simulink model "pathFollowingWithObstacleAvoidanceExample"  (R2018a)
settings: Solver=VariableStepAuto  StartTime=0.0  StopTime=inf  FixedStep=0.01  RelTol=1e-3  EnableMultiTasking=on
model workspace (MAT data in the model file):
  SL_ROS_VariableLengthArrays_MaxSizes.CommonInfo.ArrayTruncateAction = 'EmitWarning'
  SL_ROS_VariableLengthArrays_MaxSizes.MsgTypeMap = containers.Map
  SL_ROS_VariableLengthArrays_MaxSizes.MsgTypeMap.serialization.keys = {'sensor_msgs/CompressedImage', 'sensor_msgs/LaserScan'}
  SL_ROS_VariableLengthArrays_MaxSizes.MsgTypeMap.serialization.values{1}(1).PropertyName = 'Data'
  SL_ROS_VariableLengthArrays_MaxSizes.MsgTypeMap.serialization.values{1}(1).DataType = 'uint8'
  SL_ROS_VariableLengthArrays_MaxSizes.MsgTypeMap.serialization.values{1}(1).MaxLength = 10000000
  SL_ROS_VariableLengthArrays_MaxSizes.MsgTypeMap.serialization.values{1}(2).PropertyName = 'Format'
  SL_ROS_VariableLengthArrays_MaxSizes.MsgTypeMap.serialization.values{1}(2).DataType = 'uint8'
  SL_ROS_VariableLengthArrays_MaxSizes.MsgTypeMap.serialization.values{1}(2).MaxLength = 128
  SL_ROS_VariableLengthArrays_MaxSizes.MsgTypeMap.serialization.values{2}(1).PropertyName = 'Intensities'
  SL_ROS_VariableLengthArrays_MaxSizes.MsgTypeMap.serialization.values{2}(1).DataType = 'single'
  SL_ROS_VariableLengthArrays_MaxSizes.MsgTypeMap.serialization.values{2}(1).MaxLength = 4000
  SL_ROS_VariableLengthArrays_MaxSizes.MsgTypeMap.serialization.values{2}(2).PropertyName = 'Ranges'
  SL_ROS_VariableLengthArrays_MaxSizes.MsgTypeMap.serialization.values{2}(2).DataType = 'single'
  SL_ROS_VariableLengthArrays_MaxSizes.MsgTypeMap.serialization.values{2}(2).MaxLength = 4000
  SL_ROS_VariableLengthArrays_MaxSizes.MsgTypeMap.serialization.uniformity = 0
  SL_ROS_VariableLengthArrays_MaxSizes.MsgTypeMap.serialization.keyType = 'char'
  SL_ROS_VariableLengthArrays_MaxSizes.MsgTypeMap.serialization.valueType = 'any'
undefined symbols (not defined in the file or in its folder): Angular, gray, Linear
libraries: robotlib x8, robotalgslib x2, simulink x1
settings Model: Creator=The MathWorks, Inc.  LastModifiedBy=SangjunLee
settings CodeAppCC: StateflowObjectComments=on
settings GRTTargetCC: TargetLangStandard=C89/C90 (ANSI)
settings ConfigComp: CovMetricSettings=dsw  CovHtmlReporting=on  CovSaveCumulativeToWorkspaceVar=on  CovSaveSingleToWorkspaceVar=on  CovExternalEMLEnable=off

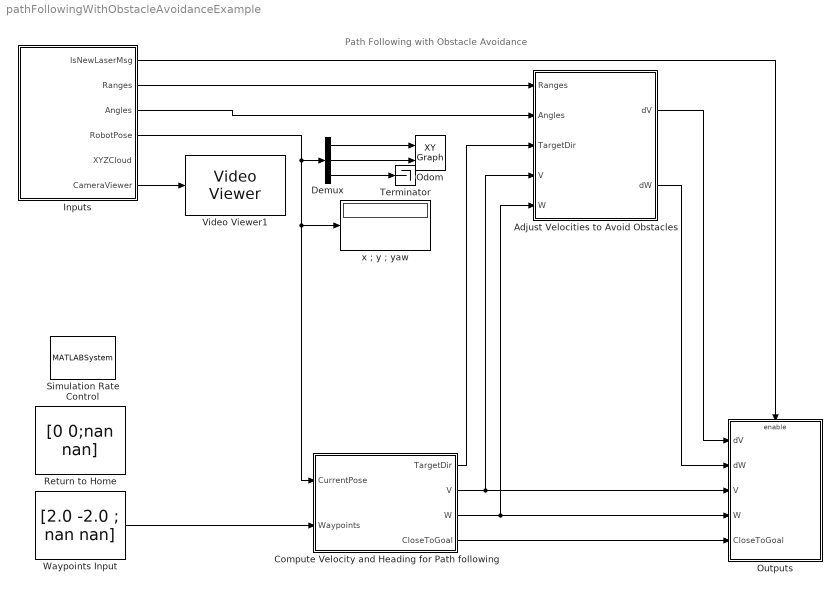
== system pathFollowingWithObstacleAvoidanceExample ==
  note: Path Following with Obstacle Avoidance
  Adjust Velocities to Avoid Obstacles : Subsystem
  Compute Velocity and Heading for Path following : Subsystem
  Demux : Demux  Outputs=3
  Inputs : Subsystem
  Odom : simulink/Sinks/XY Graph  xmin=-5  xmax=5  ymin=-5  ymax=5  st=-1
  Outputs : Subsystem
  Return to Home : Constant  Value=[0 0;nan nan]  OutDataTypeStr=double
  Simulation Rate Control : MATLABSystem  System=ExampleHelperSimulationRateControl  SampleTime=0.001
      mask Type: ExampleHelperSimulationRateControl
      mask Display: disp('Rate Control');
  Terminator : Terminator
  Video Viewer1 : VideoViewer  colormapValue=gray(256)  FigPos=[-763 152 382 198]
  Waypoints Input : Constant  Value=[2.0 -2.0 ; nan nan]  OutDataTypeStr=double
  x ; y ; yaw : Display
  wires:
  Compute Velocity and Heading for Path following/2(V) -> Adjust Velocities to Avoid Obstacles/4(V), Outputs/3(V)
  Compute Velocity and Heading for Path following/1(TargetDir) -> Adjust Velocities to Avoid Obstacles/3(TargetDir)
  Inputs/2(Ranges) -> Adjust Velocities to Avoid Obstacles/1(Ranges)
  Inputs/3(Angles) -> Adjust Velocities to Avoid Obstacles/2(Angles)
  Inputs/1(IsNewLaserMsg) -> Outputs/Enable
  Waypoints Input/1 -> Compute Velocity and Heading for Path following/2(Waypoints)
  Compute Velocity and Heading for Path following/3(W) -> Adjust Velocities to Avoid Obstacles/5(W), Outputs/4(W)
  Adjust Velocities to Avoid Obstacles/1(dV) -> Outputs/1(dV)
  Adjust Velocities to Avoid Obstacles/2(dW) -> Outputs/2(dW)
  Compute Velocity and Heading for Path following/4(CloseToGoal) -> Outputs/5(CloseToGoal)
  Inputs/4(RobotPose) -> Compute Velocity and Heading for Path following/1(CurrentPose), x ; y ; yaw/1, Demux/1
  Demux/2 -> Odom/2
  Demux/1 -> Odom/1
  Demux/3 -> Terminator/1
  Inputs/6(CameraViewer) -> Video Viewer1/1

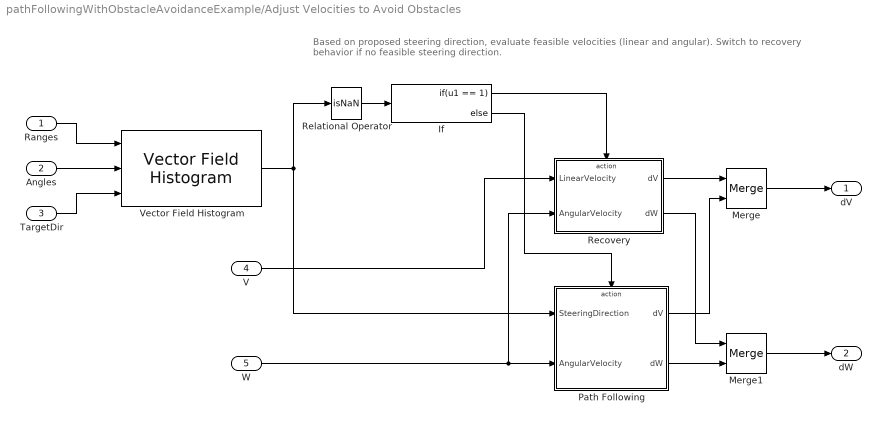
== system pathFollowingWithObstacleAvoidanceExample/Adjust Velocities to Avoid Obstacles ==
  note: Based on proposed steering direction, evaluate feasible velocities (linear and angular).
      | 				Switch to recovery behavior if no feasible steering direction.
  Ranges : Inport
  Angles : Inport  Port=2
  TargetDir : Inport  Port=3
  V : Inport  Port=4
  W : Inport  Port=5
  If : If  IfExpression=u1 == 1
  Merge : Merge
  Merge1 : Merge
  Path Following : Subsystem  TreatAsAtomicUnit=on
  Recovery : Subsystem  TreatAsAtomicUnit=on
  Relational Operator : RelationalOperator  Operator=isNaN  OutDataTypeStr=boolean  RndMeth=Simplest
  Vector Field Histogram : robotalgslib/Vector Field Histogram  NumAngularSectors=180  DistanceLimits=[ 0.05, 3 ]  HistogramThresholds=[ 3, 8 ]  RobotRadius=0.2  SafetyDistance=0.3  MinTurningRadius=0.1  SimulateUsing=Code generation  TargetDirectionWeight=5  CurrentDirectionWeight=2  PreviousDirectionWeight=2
      settings: SourceProductName=Robotics System Toolbox  SourceProductBaseCode=RO
  dV : Outport
  dW : Outport  Port=2
  wires:
  Merge1/1 -> dW/1
  V/1 -> Recovery/1(LinearVelocity)
  Vector Field Histogram/1 -> Relational Operator/1, Path Following/1(SteeringDirection)
  W/1 -> Recovery/2(AngularVelocity), Path Following/2(AngularVelocity)
  Relational Operator/1 -> If/1
  Angles/1 -> Vector Field Histogram/2
  Merge/1 -> dV/1
  TargetDir/1 -> Vector Field Histogram/3
  Ranges/1 -> Vector Field Histogram/1
  If/1 -> Recovery/Action
  If/2 -> Path Following/Action
  Recovery/2(dW) -> Merge1/1
  Path Following/2(dW) -> Merge1/2
  Recovery/1(dV) -> Merge/1
  Path Following/1(dV) -> Merge/2

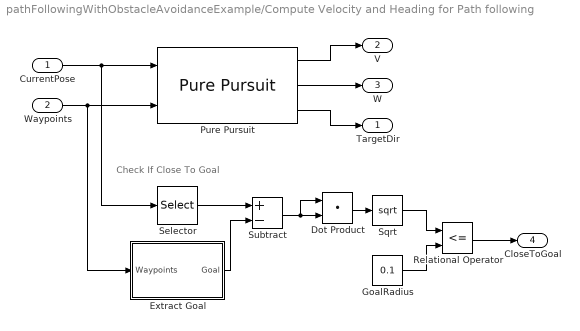
== system pathFollowingWithObstacleAvoidanceExample/Compute Velocity and Heading for Path following ==
  note: Check If Close To Goal
  CurrentPose : Inport
  Waypoints : Inport  Port=2
  " Extract Goal" : MATLAB Function  TreatAsAtomicUnit=on
  Dot Product : DotProduct  InputSameDT=on  OutDataTypeStr=Inherit: Inherit via internal rule
  GoalRadius : Constant  Value=0.1
  Pure Pursuit : robotalgslib/Pure Pursuit  DesiredLinearVelocity=0.2  MaxAngularVelocity=0.05  LookaheadDistance=0.5  TargetDirPort=on  SimulateUsing=Code generation
      settings: SourceProductName=Robotics System Toolbox  SourceProductBaseCode=RO
  Relational Operator : RelationalOperator  Operator=<=  OutDataTypeStr=boolean  RndMeth=Simplest
  Selector : Selector  InputPortWidth=3  IndexOptions=Index vector (dialog)  Indices=[1 2]  OutputSizes=1
  Sqrt : Sqrt  SaturateOnIntegerOverflow=on
  Subtract : Sum  Inputs=+-
  TargetDir : Outport
  V : Outport  Port=2
  W : Outport  Port=3
  CloseToGoal : Outport  Port=4
  wires:
  Pure Pursuit/3 -> TargetDir/1
  Pure Pursuit/2 -> W/1
  Pure Pursuit/1 -> V/1
  " Extract Goal"/1(Goal) -> Subtract/2
  Waypoints/1 -> " Extract Goal"/1(Waypoints), Pure Pursuit/2
  CurrentPose/1 -> Selector/1, Pure Pursuit/1
  Relational Operator/1 -> CloseToGoal/1
  GoalRadius/1 -> Relational Operator/2
  Selector/1 -> Subtract/1
  Dot Product/1 -> Sqrt/1
  Sqrt/1 -> Relational Operator/1
  Subtract/1 -> Dot Product/1, Dot Product/2

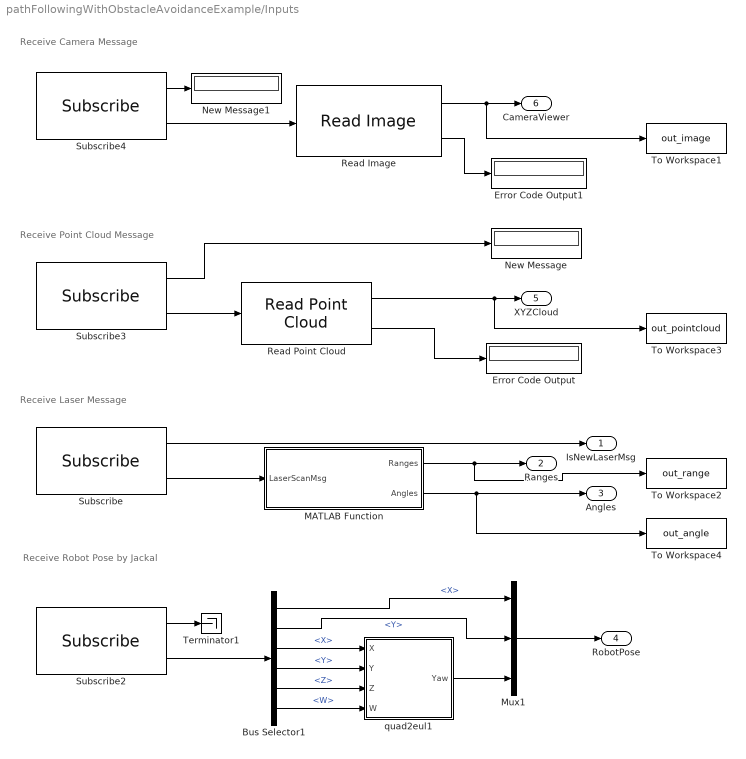
== system pathFollowingWithObstacleAvoidanceExample/Inputs ==
  note: Receive Laser Message
  note: Receive Robot Pose by Jackal
  note: Receive Point Cloud Message
  note: Receive Camera Message
  Bus Selector1 : BusSelector  OutputSignals=Pose.Pose.Position.X,Pose.Pose.Position.Y,Pose.Pose.Orientation.X,Pose.Pose.Orientation.Y,Pose.Pose.Orientation.Z,Pose.Pose.Orientation.W
  Error Code Output : Display
  Error Code Output1 : Display
  MATLAB Function : MATLAB Function  TreatAsAtomicUnit=on
  Mux1 : Mux  Inputs=3
  New Message : Display
  New Message1 : Display
  Read Image : robotlib/Read Image  SourceLibraryInfo=This block requires Robotics System Toolbox  MaximumImageSize=[720, 1280]  ImageEncoding=bgr8  ShowAlphaOutput=off  ShowErrorCodeOutput=on  VariableSizeOutputs=off
      settings: SourceProductName=Robotics System Toolbox  SourceProductBaseCode=RO
  Read Point Cloud : robotlib/Read Point Cloud  SourceLibraryInfo=This block requires Robotics System Toolbox  MaximumPointCloudSize=[ 480, 640 ]  PreserveStructure=off  ShowRGBOutput=off  ShowIntensityOutput=off  ShowErrorCodeOutput=on  VariableSizeOutputs=off
      settings: SourceProductName=Robotics System Toolbox  SourceProductBaseCode=RO
  Subscribe : robotlib/Subscribe  SourceLibraryInfo=This block requires Robotics System Toolbox  topicSource=Select from ROS network  topic=/scan  messageType=sensor_msgs/LaserScan  sampleTime=-1  messageQueueLength=1
      settings: SourceProductBaseCode=RO
  Subscribe2 : robotlib/Subscribe  SourceLibraryInfo=This block requires Robotics System Toolbox  topicSource=Select from ROS network  topic=/jackal_velocity_controller/odom  messageType=nav_msgs/Odometry  sampleTime=-1  messageQueueLength=1
      settings: SourceProductBaseCode=RO
  Subscribe3 : robotlib/Subscribe  SourceLibraryInfo=This block requires Robotics System Toolbox  topicSource=Select from ROS network  topic=/velodyne_points  messageType=sensor_msgs/PointCloud2  sampleTime=-1  messageQueueLength=1
      settings: SourceProductBaseCode=RO
  Subscribe4 : robotlib/Subscribe  SourceLibraryInfo=This block requires Robotics System Toolbox  topicSource=Select from ROS network  topic=/axis/image_raw/compressed  messageType=sensor_msgs/CompressedImage  sampleTime=-1  messageQueueLength=1
      settings: SourceProductBaseCode=RO
  Terminator1 : Terminator
  To Workspace1 : ToWorkspace  VariableName=out_image  SaveFormat=Timeseries  SampleTime=-1
  To Workspace2 : ToWorkspace  VariableName=out_range  SaveFormat=Timeseries  SampleTime=-1
  To Workspace3 : ToWorkspace  VariableName=out_pointcloud  SaveFormat=Timeseries  SampleTime=-1
  To Workspace4 : ToWorkspace  VariableName=out_angle  SaveFormat=Timeseries  SampleTime=-1
  quad2eul1 : MATLAB Function  TreatAsAtomicUnit=on
  IsNewLaserMsg : Outport
  Ranges : Outport  Port=2
  Angles : Outport  Port=3
  RobotPose : Outport  Port=4
  XYZCloud : Outport  Port=5
  CameraViewer : Outport  Port=6
  wires:
  Subscribe/2 -> MATLAB Function/1(LaserScanMsg)
  MATLAB Function/1(Ranges) -> To Workspace2/1, Ranges/1
  MATLAB Function/2(Angles) -> To Workspace4/1, Angles/1
  Subscribe/1 -> IsNewLaserMsg/1
  Bus Selector1/3 -> quad2eul1/1(X)  "<X>"
  Bus Selector1/5 -> quad2eul1/3(Z)  "<Z>"
  quad2eul1/1(Yaw) -> Mux1/3
  Bus Selector1/4 -> quad2eul1/2(Y)  "<Y>"
  Bus Selector1/2 -> Mux1/2  "<Y>"
  Subscribe2/1 -> Terminator1/1
  Bus Selector1/1 -> Mux1/1  "<X>"
  Subscribe2/2 -> Bus Selector1/1
  Bus Selector1/6 -> quad2eul1/4(W)  "<W>"
  Mux1/1 -> RobotPose/1
  Read Point Cloud/1 -> To Workspace3/1, XYZCloud/1
  Subscribe3/2 -> Read Point Cloud/1
  Subscribe3/1 -> New Message/1
  Read Point Cloud/2 -> Error Code Output/1
  Subscribe4/1 -> New Message1/1
  Subscribe4/2 -> Read Image/1
  Read Image/1 -> To Workspace1/1, CameraViewer/1
  Read Image/2 -> Error Code Output1/1

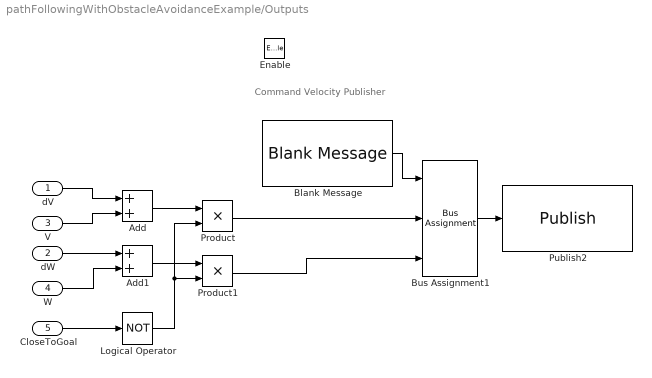
== system pathFollowingWithObstacleAvoidanceExample/Outputs ==
  note: Command Velocity Publisher
  dV : Inport
  dW : Inport  Port=2
  V : Inport  Port=3
  W : Inport  Port=4
  CloseToGoal : Inport  Port=5
  Enable : EnablePort
  Add : Sum
  Add1 : Sum
  Blank Message : robotlib/Blank Message  SourceLibraryInfo=This block requires Robotics System Toolbox  messageType=geometry_msgs/Twist  SampleTime=inf
      settings: SourceProductBaseCode=RO
  Bus Assignment1 : BusAssignment  DialogController=Simulink.DDGSource_BusAssignment  AssignedSignals=Linear.X,Angular.Z
  Logical Operator : Logic  Operator=NOT  AllPortsSameDT=off  OutDataTypeStr=boolean
  Product : Product
  Product1 : Product
  Publish2 : robotlib/Publish  SourceLibraryInfo=This block requires Robotics System Toolbox  topicSource=Select from ROS network  topic=/jackal_velocity_controller/cmd_vel  messageType=geometry_msgs/Twist  messageQueueLength=105
      settings: SourceProductBaseCode=RO
  wires:
  V/1 -> Add/2
  W/1 -> Add1/2
  dV/1 -> Add/1
  dW/1 -> Add1/1
  CloseToGoal/1 -> Logical Operator/1
  Add/1 -> Product/1
  Add1/1 -> Product1/1
  Product1/1 -> Bus Assignment1/3
  Product/1 -> Bus Assignment1/2
  Blank Message/1 -> Bus Assignment1/1
  Bus Assignment1/1 -> Publish2/1
  Logical Operator/1 -> Product1/2, Product/2

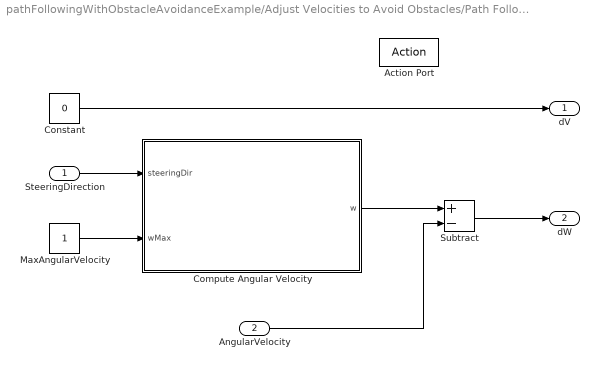
== system pathFollowingWithObstacleAvoidanceExample/Adjust Velocities to Avoid Obstacles/Path Following ==
  SteeringDirection : Inport
  AngularVelocity : Inport  Port=2
  Action Port : ActionPort  ActionType=else
  Compute Angular Velocity : MATLAB Function  TreatAsAtomicUnit=on
  Constant : Constant  Value=0
  MaxAngularVelocity : Constant
  Subtract : Sum  Inputs=+-
  dV : Outport
  dW : Outport  Port=2
  wires:
  Constant/1 -> dV/1
  MaxAngularVelocity/1 -> Compute Angular Velocity/2(wMax)
  SteeringDirection/1 -> Compute Angular Velocity/1(steeringDir)
  Subtract/1 -> dW/1
  Compute Angular Velocity/1(w) -> Subtract/1
  AngularVelocity/1 -> Subtract/2

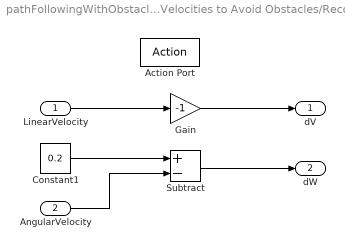
== system pathFollowingWithObstacleAvoidanceExample/Adjust Velocities to Avoid Obstacles/Recovery ==
  LinearVelocity : Inport
  AngularVelocity : Inport  Port=2
  Action Port : ActionPort  ActionType=then
  Constant1 : Constant  Value=0.2
  Gain : Gain  Gain=-1
  Subtract : Sum  Inputs=+-
  dV : Outport
  dW : Outport  Port=2
  wires:
  LinearVelocity/1 -> Gain/1
  Gain/1 -> dV/1
  Constant1/1 -> Subtract/1
  AngularVelocity/1 -> Subtract/2
  Subtract/1 -> dW/1

== matlab function pathFollowingWithObstacleAvoidanceExample/Inputs/quad2eul1 ==
  data: X input; Yaw output; Y input; Z input; W input
function Yaw = quat2eulBlk(X, Y, Z, W)
%#codegen

eularAngles = quat2eul([W, X, Y, Z]);
Yaw = eularAngles(1);

== matlab function pathFollowingWithObstacleAvoidanceExample/Inputs/MATLAB Function ==
  data: LaserScanMsg input; Ranges output; Angles output
function [Ranges, Angles] = ExtractRangeData(LaserScanMsg)
%#codegen

% Extract Range information
Ranges = double(LaserScanMsg.Ranges);

% Construct Angles vector using AngleMin and AngleIncrement from sensor
% reading.
angMin = double(LaserScanMsg.AngleMin);
angIncrement = double(LaserScanMsg.AngleIncrement);

numReadings = numel(Ranges);
rawAngles = angMin + (0:numReadings-1)' * angIncrement;

% Wrap the angles to the (-pi,pi] interval.
Angles = robotics.internal.wrapToPi(double(rawAngles));

== matlab function pathFollowingWithObstacleAvoidanceExample/Compute Velocity and Heading for Path following/ Extract Goal ==
  data: Waypoints input; Goal output
function Goal = extractGoal(Waypoints)
%#codegen
b = isnan(Waypoints);
[rows,~] = find(b);
ridx = setdiff(1:size(Waypoints,1), sort(rows));
Goal = [Waypoints(ridx(end), 1) Waypoints(ridx(end), 2)];

== matlab function pathFollowingWithObstacleAvoidanceExample/Adjust Velocities to Avoid Obstacles/Path Following/Compute Angular Velocity ==
  data: steeringDir input; w output; wMax input
function w = exampleHelperComputeAngularVelocity(steeringDir, wMax)
%EXAMPLEHELPERCOMPUTEANGULARVELOCITY Compute angular velocity
%   W = exampleHelperComputeAngularVelocity(STEERINGDIR)
%   returns the angular velocity W for a differential drive robot in radians
%   per second for a given steering direction STEERINGDIR in the robot's
%   coordinate frame in radians.
%
%   W = exampleHelperComputeAngularVelocity(STEERINGDIR, WMAX)
%   returns the angular velocity W for a differential drive robot in radians
%   per second for a given steering direction STEERINGDIR in the robot's
%   coordinate frame in radians and maximum angular velocity WMAX in
%   radians per second. The output angular velocity is saturated based on
%   the WMAX.
%
%   Example:
%       
%       w = exampleHelperComputeAngularVelocity(0.2, 1);

% Copyright 2015 The MathWorks, Inc.

%#codegen
%#ok<*EMCA>

% Allow variable input arguments
if nargin == 1   
    wMax = inf;
end

validateattributes(steeringDir, {'double'},{'real'},...
    'exampleHelperComputeAngularVelocity', 'STEERINGDIR', 1);
validateattributes(wMax, {'double'},{'real', 'positive'},...
    'exampleHelperComputeAngularVelocity', 'WMAX', 2);

% Computing in robot's coordinate frame
curPose = [0 0 0];

% The following computation is similar to robotics.PurePursuit
lookaheadPoint = [cos(steeringDir), sin(steeringDir)];
slope = atan2((lookaheadPoint(2) - curPose(2)), ...
    (lookaheadPoint(1) - curPose(1)));
alpha = angdiff(curPose(3), slope);

% Angular velocity command for a differential drive robot is
% equal to the desired curvature to be followed by the robot.

w = (2*sin(alpha));

% Pick a constant rotation when robot is facing in the opposite
% direction of the path
if abs(abs(alpha) - pi) < 1e-12
    w = sign(w)*1;
end

if abs(w) > wMax
    w = sign(w)*wMax;
end

end
